simulink model "Bidirectional_DC_DC_COnverter"  (R2023a)
settings: Solver=VariableStepAuto  StartTime=0.0  StopTime=0.01  RelTol=1e-3
undefined symbols (not defined in the file or in its folder): Hydride, Metal, Nickel
libraries: spsSeriesRLCBranchLib x3, spsBatteryLib x2, spsMosfetLib x2, spsVoltageMeasurementLib x2, simulink x1, sps_lib x1
settings Model: Creator=Lenovo  LastModifiedBy=Lenovo

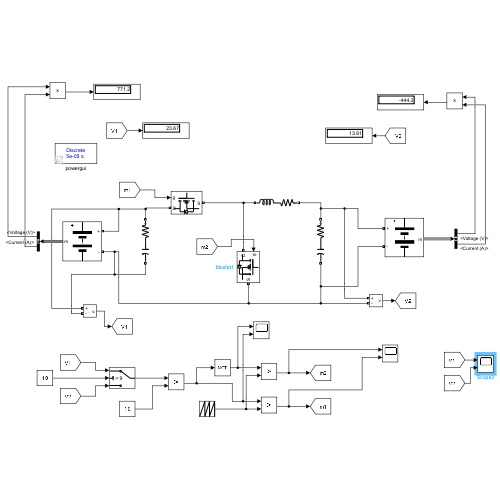
[thumbnail: Simulink's stored preview of the top-level diagram]
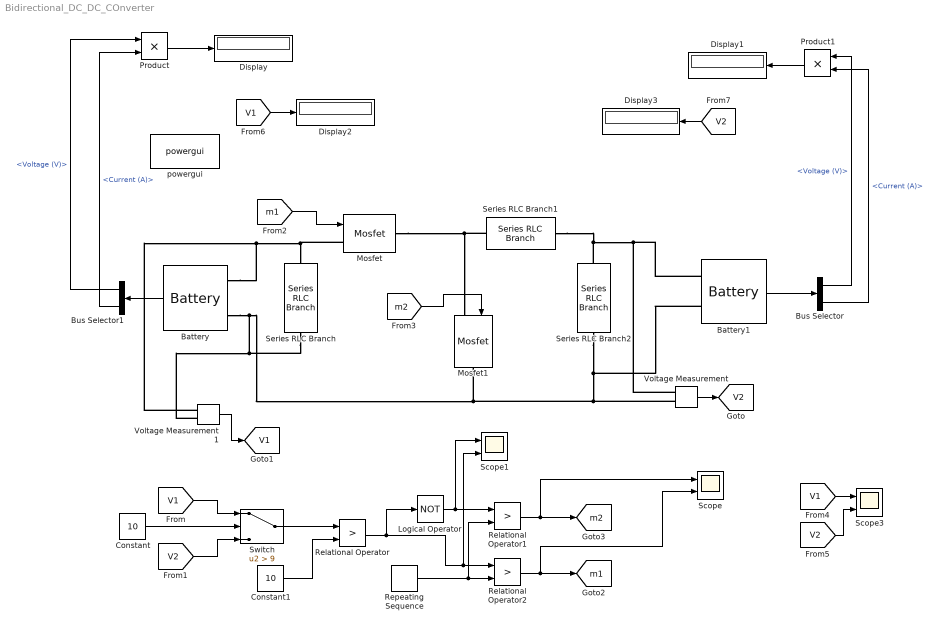
== system Bidirectional_DC_DC_COnverter ==
  Battery : spsBatteryLib/Battery  BatType=Nickel-Metal-Hydride  ShowTempParam=off  ThermalPreset=no  ShowAgeParam=off  NomV=24  NomQ=6.5  SOC=20  Batt_Tr=0.5  PresetModel=on  MaxQ=7  MinV=18  FullV=28.2712  Dis_rate=1.3  R=0.036923  Normal_OP=6.25  expZone="[26.0339          1.3]"  current=[6.5 13 32.5]  Units=Time  Tci=20  NomT=20  T2=-30  MaxQ2=4.8  FullV2=7.1  Normal_OP2=5.655  expZone2="[6.58           1]"  Rca=0.6  ti=2000  Dp=0  Neq0=0  Tsim=1e6  Ta1=25  Qeol=5.4*0.9  Reol=0.013333*1.2  Char_age=[2.3478, 3]  Dis_age=[2.3478, 10]  N1=1500  N2=10500  N3=1000  N4=1400  Ta2=45  N5=950
  Battery1 : spsBatteryLib/Battery  BatType=Nickel-Metal-Hydride  ShowTempParam=off  ThermalPreset=no  ShowAgeParam=off  NomV=12  NomQ=6.5  SOC=60  Batt_Tr=0.5  PresetModel=on  MaxQ=7  MinV=9  FullV=14.1356  Dis_rate=1.3  R=0.018462  Normal_OP=6.25  expZone="[13.0169          1.3]"  current=[6.5 13 32.5]  Units=Time  Tci=20  NomT=20  T2=-30  MaxQ2=4.8  FullV2=7.1  Normal_OP2=5.655  expZone2="[6.58           1]"  Rca=0.6  ti=2000  Dp=0  Neq0=0  Tsim=1e6  Ta1=25  Qeol=5.4*0.9  Reol=0.013333*1.2  Char_age=[2.3478, 3]  Dis_age=[2.3478, 10]  N1=1500  N2=10500  N3=1000  N4=1400  Ta2=45  N5=950
  Bus Selector : BusSelector  OutputSignals=Voltage (V),Current (A)
  Bus Selector1 : BusSelector  OutputSignals=Voltage (V),Current (A)
  Constant : Constant  Value=10
  Constant1 : Constant  Value=10
  Display{,1..3} (4 alike) : Display
  Logical Operator : Logic  Operator=NOT  AllPortsSameDT=off  OutDataTypeStr=boolean
  Mosfet : spsMosfetLib/Mosfet  Ron=0.1  Lon=0  Rd=0.01  Vfd=0  IC=0  Rs=1e5  Cs=inf  Measurements=off
  Mosfet1 : spsMosfetLib/Mosfet  Ron=0.1  Lon=0  Rd=0.01  Vfd=0  IC=0  Rs=1e5  Cs=inf  Measurements=off
  Product : Product
  Product1 : Product
  Relational Operator : RelationalOperator  Operator=>  OutDataTypeStr=boolean  RndMeth=Simplest  InputSameDT=off
  Relational Operator1 : RelationalOperator  Operator=>  OutDataTypeStr=boolean  RndMeth=Simplest  InputSameDT=off
  Relational Operator2 : RelationalOperator  Operator=>  OutDataTypeStr=boolean  RndMeth=Simplest  InputSameDT=off
  Repeating Sequence : simulink/Sources/Repeating Sequence  rep_seq_t=[0 0.00005]  rep_seq_y=[0 1]
  Scope : Scope  NumInputPorts=2
  Scope1 : Scope  NumInputPorts=2
  Scope3 : Scope  NumInputPorts=2
  Series RLC Branch : spsSeriesRLCBranchLib/Series RLC Branch  LConnTagsString=__new0  RConnTagsString=__new0  BranchType=RC  Resistance=0.1  Inductance=1e-3  SetiL0=off  InitialCurrent=0  Capacitance=2000e-6  Setx0=off  InitialVoltage=0  Measurements=None
  Series RLC Branch1 : spsSeriesRLCBranchLib/Series RLC Branch  LConnTagsString=__new0  RConnTagsString=__new0  BranchType=RL  Resistance=0.2  Inductance=1e-3  SetiL0=off  InitialCurrent=0  Capacitance=1e-6  Setx0=off  InitialVoltage=0  Measurements=None
  Series RLC Branch2 : spsSeriesRLCBranchLib/Series RLC Branch  LConnTagsString=__new0  RConnTagsString=__new0  BranchType=RC  Resistance=0.1  Inductance=1e-3  SetiL0=off  InitialCurrent=0  Capacitance=2000e-6  Setx0=off  InitialVoltage=0  Measurements=None
  Switch : Switch  Criteria=u2 > Threshold  Threshold=9  SaturateOnIntegerOverflow=off  InputSameDT=off
  Voltage Measurement : spsVoltageMeasurementLib/Voltage Measurement  PhasorSimulation=off  OutputType=Complex  PSBequivalent=0
  Voltage Measurement1 : spsVoltageMeasurementLib/Voltage Measurement  PhasorSimulation=off  OutputType=Complex  PSBequivalent=0
  powergui : sps_lib/powergui  Priority=1  SimulationMode=Discrete  SampleTime=50e-6  frequency=60  Iterations=50  frequencyindice=0  Pbase=100e6  ErrMax=1e-4  UnitsV=kV  UnitsW=MW  buscounter=0  FunctionMessages=off  echomessages=off  EnableUseOfTLC=off  CurrentSourceSwitches=off  DisableSnubberDevices=off  DisableRonSwitches=off  DisableVfSwitches=off  DisplayEquations=off  AutomaticDiscreteSolvers=off  SolverType=Tustin/Backward Euler (TBE)  Interpol=off  ExternalGateDelay=off  methode=off  Ts=100  x0status=blocks  SPID=on  SwTol=0  HookPort=off  NonlinearTolerance=1e-4  nMaxIteration=100  ContinueOnMaxIteration=off  RestoreLinks=warning  ResistiveCurrentMeasurement=off  Frange=[0:2:500]  Ylog=off  Xlog=on  ShowGrid=off  save=off  variable=ZData  structure=0  ZoomFFT=off  StartTime=0.0  cycles=1  DisplayStyle=1  fundamental=60  FreqAxis=off  MaxFrequency=1000  frequencyindicesteady=1  RmsSteady=1  display=off
  tag scope: V1=global, V2=global, m1=global, m2=global
  wires:
  Battery1/1 -> Bus Selector/1
  Bus Selector/1 -> Product1/1  "<Voltage (V)>"
  Battery/1 -> Bus Selector1/1
  Bus Selector1/1 -> Product/1  "<Voltage (V)>"
  Bus Selector1/2 -> Product/2  "<Current (A)>"
  Product/1 -> Display/1
  Voltage Measurement/1 -> [V2]
  Voltage Measurement1/1 -> [V1]
  [V1] -> Switch/1
  [V2] -> Switch/3
  Constant/1 -> Switch/2
  Switch/1 -> Relational Operator/1
  Constant1/1 -> Relational Operator/2
  Logical Operator/1 -> Scope1/1, Relational Operator1/1
  Relational Operator/1 -> Logical Operator/1, Scope1/2, Relational Operator2/1
  Repeating Sequence/1 -> Relational Operator1/2, Relational Operator2/2
  Relational Operator1/1 -> [m2], Scope/1
  Relational Operator2/1 -> Scope/2, [m1]
  [m2] -> Mosfet1/1
  [m1] -> Mosfet/1
  Bus Selector/2 -> Product1/2  "<Current (A)>"
  Product1/1 -> Display1/1
  [V1] -> Scope3/1
  [V2] -> Scope3/2
  [V1] -> Display2/1
  [V2] -> Display3/1
  connections:
  Battery/LConn1 -- Series RLC Branch/LConn1 -- Mosfet/LConn1 -- Voltage Measurement1/LConn1
  Series RLC Branch2/LConn1 -- Series RLC Branch1/LConn1 -- Voltage Measurement/LConn1 -- Battery1/LConn1
  Series RLC Branch2/RConn1 -- Battery1/LConn2 -- Voltage Measurement/LConn2 -- Series RLC Branch/RConn1 -- Voltage Measurement1/LConn2 -- Battery/LConn2 -- Mosfet1/RConn1
  Mosfet/RConn1 -- Mosfet1/LConn1 -- Series RLC Branch1/RConn1
